simulink subsystem "Test_Outputs"  (R2024b)
settings: Solver=VariableStepAuto  StartTime=0.0  StopTime=10.0  RelTol=1e-3
settings Model: Creator=schwmaxi  LastModifiedBy=schwmaxi

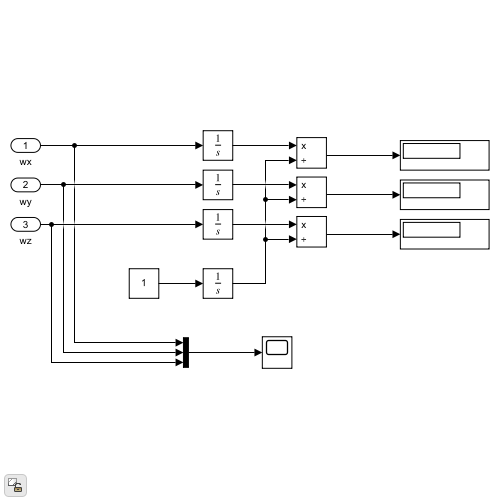
[thumbnail: Simulink's stored preview of the top-level diagram]
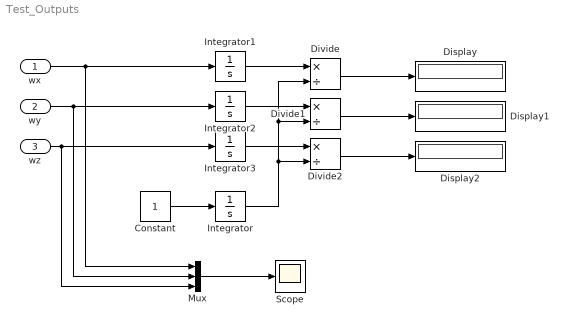
== system Test_Outputs ==
  wx : Inport
  wy : Inport  Port=2
  wz : Inport  Port=3
  Constant : Constant
  Display : Display
  Display1 : Display
  Display2 : Display
  Divide : Product  Inputs=*/
  Divide1 : Product  Inputs=*/
  Divide2 : Product  Inputs=*/
  Integrator{,1..3} (4 alike) : Integrator
  Mux : Mux  Inputs=3
  Scope : Scope
  wires:
  Integrator/1 -> Divide2/2, Divide1/2, Divide/2
  Divide2/1 -> Display2/1
  Divide/1 -> Display/1
  Mux/1 -> Scope/1
  Divide1/1 -> Display1/1
  Integrator2/1 -> Divide1/1
  Integrator3/1 -> Divide2/1
  Constant/1 -> Integrator/1
  Integrator1/1 -> Divide/1
  wx/1 -> Integrator1/1, Mux/1
  wy/1 -> Integrator2/1, Mux/2
  wz/1 -> Integrator3/1, Mux/3
